simulink model "FIS_Controller"  (R2020b)
settings: Solver=VariableStepAuto  StartTime=0.0  StopTime=200  RelTol=1e-3
libraries: simulink x1, fuzblock x1
settings Model: Creator=smsmt  LastModifiedBy=smsmt

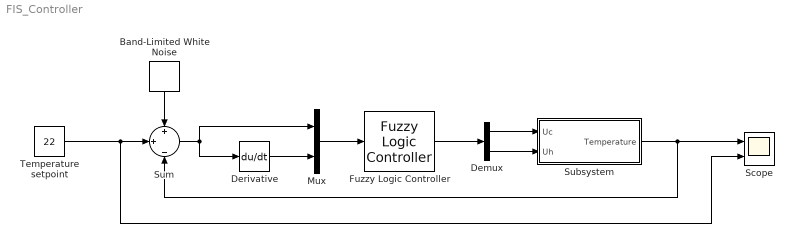
== system FIS_Controller ==
  Band-Limited White Noise : simulink/Sources/Band-Limited White Noise  Cov=[0]  Ts=0.1  seed=[23341]
  Demux : Demux  Outputs=2
  Derivative : Derivative
  Fuzzy Logic Controller : fuzblock/Fuzzy Logic  Controller  FIS=FIS  OutputSampleNumber=101  DataType=double  FuzzifiedInputs=off  RuleFiringStrengths=off  RuleOutputs=off  AggregatedOutputs=off  SimulateUsing=Interpreted execution  OutOfRangeInputValueMessage=warning  NoRuleFiredMessage=warning  EmptyOutputFuzzySetMessage=warning
  Mux : Mux  Inputs=2
  Scope : Scope  NumInputPorts=2
  Subsystem : Subsystem
  Sum : Sum  Inputs=+|+|-
  Temperature setpoint : Constant  Value=22
  wires:
  Subsystem/1(Temperature) -> Sum/3, Scope/1
  Demux/1 -> Subsystem/1(Uc)
  Fuzzy Logic Controller/1 -> Demux/1
  Demux/2 -> Subsystem/2(Uh)
  Mux/1 -> Fuzzy Logic Controller/1
  Derivative/1 -> Mux/2
  Sum/1 -> Derivative/1, Mux/1
  Temperature setpoint/1 -> Scope/2, Sum/2
  Band-Limited White Noise/1 -> Sum/1

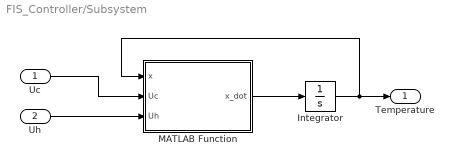
== system FIS_Controller/Subsystem ==
  Uc : Inport
  Uh : Inport  Port=2
  Integrator : Integrator
  MATLAB Function : MATLAB Function  TreatAsAtomicUnit=on
  Temperature : Outport
  wires:
  Integrator/1 -> Temperature/1, MATLAB Function/1(x)
  MATLAB Function/1(x_dot) -> Integrator/1
  Uc/1 -> MATLAB Function/2(Uc)
  Uh/1 -> MATLAB Function/3(Uh)

== matlab function FIS_Controller/Subsystem/MATLAB Function ==
  data: x input; Uc input; Uh input; x_dot output
function x_dot = fcn(x, Uc, Uh)
    x_dot = -0.1 * (x - 17) - Uc + Uh;
